simulink model "PhysicalEverSimmer"  (R2026a)
settings: Solver=VariableStepAuto  StopTime=14400
undefined symbols (not defined in the file): ES_PackRate_bph, ES_PrepRate_bph, ES_QCRate_bph, ES_Resupply_bph, Fault_T_Cell1, Fault_T_Cell2, Fault_T_Cell3, Recipe_Block_s, Recipe_Count, Resupply_Cutoff_T, Transport_Latency_s, Transport_Rate_bph
(part 1 of 2)
settings Model: DataDictionary=PhysicalEverSimmerData.sldd  Creator=sarah  LastModifiedBy=sdagen

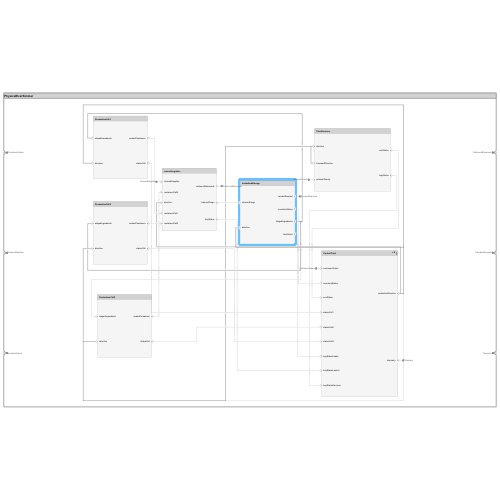
[thumbnail: Simulink's stored preview of the top-level diagram]
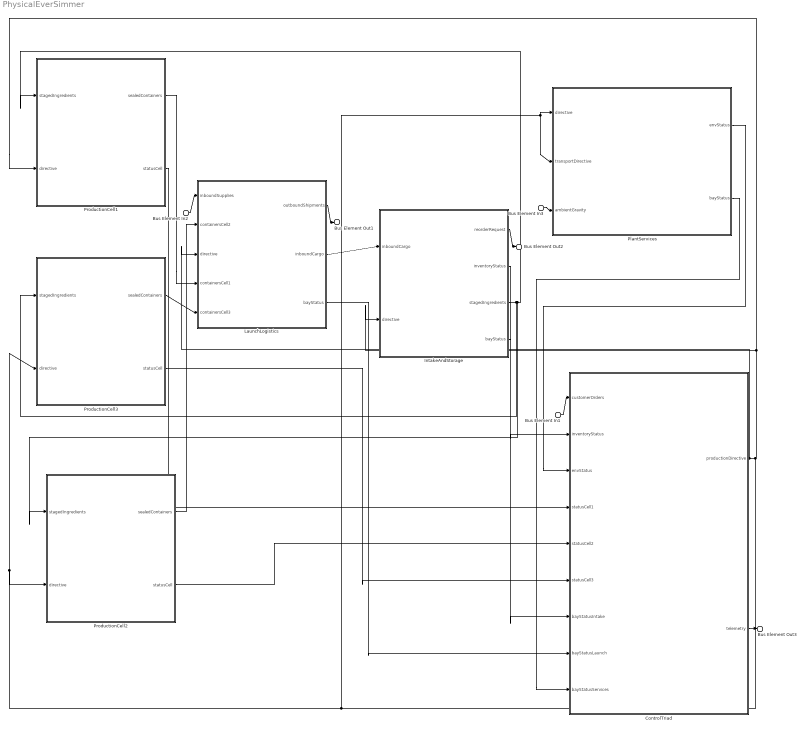
== system PhysicalEverSimmer ==
  Bus Element In1 : Inport  PortName=CustomerOrders
  Bus Element In2 : Inport  Port=2  PortName=InboundSupplies
  Bus Element In3 : Inport  Port=3  PortName=AmbientGravity
  ControlTriad : Subsystem
      settings: PortSchema="{\"entries\":[{\"content\":{\"headerSize\":26,\"margin\":15,\"minimumSpacing\":25,\"sides\":[{\"content\":{\"connectorIds\":[\"In1\",\"In2\",\"In3\",\"In4\",\"In5\",\"In6\",\"In7\",\"In8\",\"In9\"]},\"type\":\"ConnectorPlacement.EquallySpacedRectSide\",\"uuid\":\"f830f98a-8e8b-4468-adf4-d6eab644987f\"},{\"content\":{\"connectorIds\":[\"Out1\",\"Out2\"],\"side\":\"RIGHT\"},\"type\":\"ConnectorPlacement.EquallySpacedRectSide\",\"uuid\":\"7e0d0116-b3ba-4668-b638-30d0f54ba087\"},{\"content\":{\"side\":\"TOP\"},\"type\":\"ConnectorPlacement.EquallySpacedRectSide\",\"uuid\":\"7b4146d3-46d2-45ca-8c34-b106f0d8cedd\"}]},\"type\":\"ConnectorPlacement.EquallySpacedConnector\",\"uuid\":\"3d911b2d-a78f-42ea-b869-5e09982d9f54\"}],\"packageUris\":[\"http://schema.mathworks.com/mf0/Connector/R2020b\"],\"version\":\"1.0\"}"
  IntakeAndStorage : Subsystem
      settings: PortSchema="{\"entries\":[{\"content\":{\"headerSize\":26,\"margin\":15,\"minimumSpacing\":25,\"sides\":[{\"content\":{\"connectorIds\":[\"In1\",\"In2\"]},\"type\":\"ConnectorPlacement.EquallySpacedRectSide\",\"uuid\":\"3a94c7fc-0b9e-4df5-a2de-1d2483378dcb\"},{\"content\":{\"connectorIds\":[\"Out1\",\"Out2\",\"Out3\",\"Out4\"],\"side\":\"RIGHT\"},\"type\":\"ConnectorPlacement.EquallySpacedRectSide\",\"uuid\":\"607e1f04-41cc-4c9a-b401-96cdf33819d0\"},{\"content\":{\"side\":\"TOP\"},\"type\":\"ConnectorPlacement.EquallySpacedRectSide\",\"uuid\":\"2ee07fc7-54c6-4cee-9888-3f37ad01f332\"}]},\"type\":\"ConnectorPlacement.EquallySpacedConnector\",\"uuid\":\"f91f3af9-eaeb-4625-ae6e-5ceb7fb8b64c\"}],\"packageUris\":[\"http://schema.mathworks.com/mf0/Connector/R2020b\"],\"version\":\"1.0\"}"
  LaunchLogistics : Subsystem
      settings: PortSchema="{\"entries\":[{\"content\":{\"headerSize\":26,\"margin\":15,\"minimumSpacing\":25,\"sides\":[{\"content\":{\"connectorIds\":[\"In1\",\"In2\",\"In3\",\"In4\",\"In5\"]},\"type\":\"ConnectorPlacement.EquallySpacedRectSide\",\"uuid\":\"3a94c7fc-0b9e-4df5-a2de-1d2483378dcb\"},{\"content\":{\"connectorIds\":[\"Out1\",\"Out2\",\"Out3\"],\"side\":\"RIGHT\"},\"type\":\"ConnectorPlacement.EquallySpacedRectSide\",\"uuid\":\"607e1f04-41cc-4c9a-b401-96cdf33819d0\"},{\"content\":{\"side\":\"TOP\"},\"type\":\"ConnectorPlacement.EquallySpacedRectSide\",\"uuid\":\"2ee07fc7-54c6-4cee-9888-3f37ad01f332\"}]},\"type\":\"ConnectorPlacement.EquallySpacedConnector\",\"uuid\":\"f91f3af9-eaeb-4625-ae6e-5ceb7fb8b64c\"}],\"packageUris\":[\"http://schema.mathworks.com/mf0/Connector/R2020b\"],\"version\":\"1.0\"}"
  PlantServices : Subsystem
      settings: PortSchema="{\"entries\":[{\"content\":{\"headerSize\":26,\"margin\":15,\"minimumSpacing\":25,\"sides\":[{\"content\":{\"connectorIds\":[\"In1\",\"In2\",\"In3\"]},\"type\":\"ConnectorPlacement.EquallySpacedRectSide\",\"uuid\":\"3a94c7fc-0b9e-4df5-a2de-1d2483378dcb\"},{\"content\":{\"connectorIds\":[\"Out1\",\"Out2\"],\"side\":\"RIGHT\"},\"type\":\"ConnectorPlacement.EquallySpacedRectSide\",\"uuid\":\"607e1f04-41cc-4c9a-b401-96cdf33819d0\"},{\"content\":{\"side\":\"TOP\"},\"type\":\"ConnectorPlacement.EquallySpacedRectSide\",\"uuid\":\"2ee07fc7-54c6-4cee-9888-3f37ad01f332\"}]},\"type\":\"ConnectorPlacement.EquallySpacedConnector\",\"uuid\":\"f91f3af9-eaeb-4625-ae6e-5ceb7fb8b64c\"}],\"packageUris\":[\"http://schema.mathworks.com/mf0/Connector/R2020b\"],\"version\":\"1.0\"}"
  ProductionCell1 : Subsystem
      settings: PortSchema="{\"entries\":[{\"content\":{\"headerSize\":26,\"margin\":15,\"minimumSpacing\":25,\"sides\":[{\"content\":{\"connectorIds\":[\"In1\",\"In2\"]},\"type\":\"ConnectorPlacement.EquallySpacedRectSide\",\"uuid\":\"f830f98a-8e8b-4468-adf4-d6eab644987f\"},{\"content\":{\"connectorIds\":[\"Out1\",\"Out2\"],\"side\":\"RIGHT\"},\"type\":\"ConnectorPlacement.EquallySpacedRectSide\",\"uuid\":\"7e0d0116-b3ba-4668-b638-30d0f54ba087\"},{\"content\":{\"side\":\"TOP\"},\"type\":\"ConnectorPlacement.EquallySpacedRectSide\",\"uuid\":\"7b4146d3-46d2-45ca-8c34-b106f0d8cedd\"}]},\"type\":\"ConnectorPlacement.EquallySpacedConnector\",\"uuid\":\"3d911b2d-a78f-42ea-b869-5e09982d9f54\"}],\"packageUris\":[\"http://schema.mathworks.com/mf0/Connector/R2020b\"],\"version\":\"1.0\"}"
  ProductionCell2 : Subsystem
      settings: PortSchema="{\"entries\":[{\"content\":{\"headerSize\":26,\"margin\":15,\"minimumSpacing\":25,\"sides\":[{\"content\":{\"connectorIds\":[\"In1\",\"In2\"]},\"type\":\"ConnectorPlacement.EquallySpacedRectSide\",\"uuid\":\"f830f98a-8e8b-4468-adf4-d6eab644987f\"},{\"content\":{\"connectorIds\":[\"Out1\",\"Out2\"],\"side\":\"RIGHT\"},\"type\":\"ConnectorPlacement.EquallySpacedRectSide\",\"uuid\":\"7e0d0116-b3ba-4668-b638-30d0f54ba087\"},{\"content\":{\"side\":\"TOP\"},\"type\":\"ConnectorPlacement.EquallySpacedRectSide\",\"uuid\":\"7b4146d3-46d2-45ca-8c34-b106f0d8cedd\"}]},\"type\":\"ConnectorPlacement.EquallySpacedConnector\",\"uuid\":\"3d911b2d-a78f-42ea-b869-5e09982d9f54\"}],\"packageUris\":[\"http://schema.mathworks.com/mf0/Connector/R2020b\"],\"version\":\"1.0\"}"
  ProductionCell3 : Subsystem
      settings: PortSchema="{\"entries\":[{\"content\":{\"headerSize\":26,\"margin\":15,\"minimumSpacing\":25,\"sides\":[{\"content\":{\"connectorIds\":[\"In1\",\"In2\"]},\"type\":\"ConnectorPlacement.EquallySpacedRectSide\",\"uuid\":\"f830f98a-8e8b-4468-adf4-d6eab644987f\"},{\"content\":{\"connectorIds\":[\"Out1\",\"Out2\"],\"side\":\"RIGHT\"},\"type\":\"ConnectorPlacement.EquallySpacedRectSide\",\"uuid\":\"7e0d0116-b3ba-4668-b638-30d0f54ba087\"},{\"content\":{\"side\":\"TOP\"},\"type\":\"ConnectorPlacement.EquallySpacedRectSide\",\"uuid\":\"7b4146d3-46d2-45ca-8c34-b106f0d8cedd\"}]},\"type\":\"ConnectorPlacement.EquallySpacedConnector\",\"uuid\":\"3d911b2d-a78f-42ea-b869-5e09982d9f54\"}],\"packageUris\":[\"http://schema.mathworks.com/mf0/Connector/R2020b\"],\"version\":\"1.0\"}"
  Bus Element Out1 : Outport  PortName=OutboundShipments
  Bus Element Out2 : Outport  Port=2  PortName=ReorderRequests
  Bus Element Out3 : Outport  Port=3  PortName=Telemetry
  wires:
  Bus Element In2/1 -> LaunchLogistics/1(inboundSupplies)
  ProductionCell2/2(statusCell) -> ControlTriad/5(statusCell2)
  LaunchLogistics/1(outboundShipments) -> Bus Element Out1/1
  ProductionCell2/1(sealedContainers) -> LaunchLogistics/2(containersCell2)
  ProductionCell1/1(sealedContainers) -> LaunchLogistics/4(containersCell1)
  ProductionCell1/2(statusCell) -> ControlTriad/4(statusCell1)
  ProductionCell3/1(sealedContainers) -> LaunchLogistics/5(containersCell3)
  IntakeAndStorage/3(stagedIngredients) -> ProductionCell2/1(stagedIngredients), ProductionCell1/1(stagedIngredients), ProductionCell3/1(stagedIngredients)
  ProductionCell3/2(statusCell) -> ControlTriad/6(statusCell3)
  LaunchLogistics/2(inboundCargo) -> IntakeAndStorage/1(inboundCargo)
  LaunchLogistics/3(bayStatus) -> ControlTriad/8(bayStatusLaunch)
  Bus Element In3/1 -> PlantServices/3(ambientGravity)
  Bus Element In1/1 -> ControlTriad/1(customerOrders)
  IntakeAndStorage/1(reorderRequest) -> Bus Element Out2/1
  IntakeAndStorage/2(inventoryStatus) -> ControlTriad/2(inventoryStatus)
  IntakeAndStorage/4(bayStatus) -> ControlTriad/7(bayStatusIntake)
  PlantServices/1(envStatus) -> ControlTriad/3(envStatus)
  PlantServices/2(bayStatus) -> ControlTriad/9(bayStatusServices)
  ControlTriad/1(productionDirective) -> PlantServices/2(transportDirective), PlantServices/1(directive), ProductionCell3/2(directive), ProductionCell2/2(directive), IntakeAndStorage/2(directive), ProductionCell1/2(directive), LaunchLogistics/3(directive)
  ControlTriad/2(telemetry) -> Bus Element Out3/1

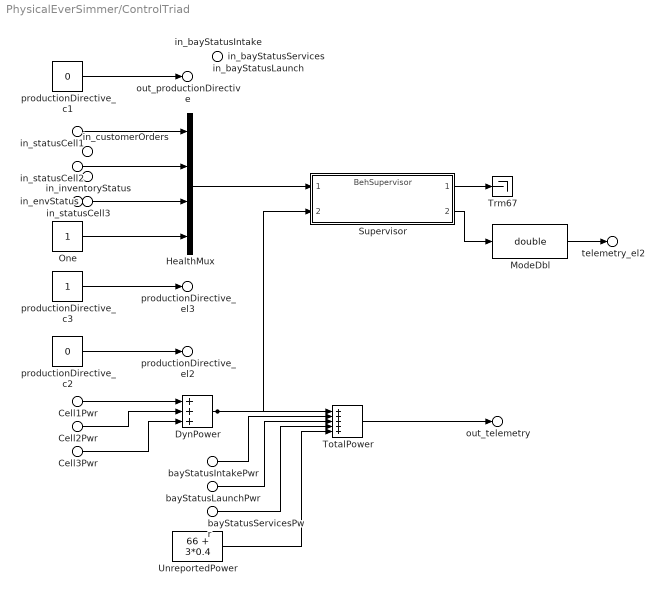
== system PhysicalEverSimmer/ControlTriad ==
  in_customerOrders : Inport  PortName=customerOrders
  in_inventoryStatus : Inport  Port=2  PortName=inventoryStatus
  in_envStatus : Inport  Port=3  PortName=envStatus
  Cell1Pwr : Inport  Port=4  PortName=statusCell1  Element=power_kW
  in_statusCell1 : Inport  Port=4  PortName=statusCell1  Element=health
  Cell2Pwr : Inport  Port=5  PortName=statusCell2  Element=power_kW
  in_statusCell2 : Inport  Port=5  PortName=statusCell2  Element=health
  Cell3Pwr : Inport  Port=6  PortName=statusCell3  Element=power_kW
  in_statusCell3 : Inport  Port=6  PortName=statusCell3  Element=health
  in_bayStatusIntake : Inport  Port=7  PortName=bayStatusIntake
  bayStatusIntakePwr : Inport  Port=7  PortName=bayStatusIntake  Element=power_kW
  in_bayStatusLaunch : Inport  Port=8  PortName=bayStatusLaunch
  bayStatusLaunchPwr : Inport  Port=8  PortName=bayStatusLaunch  Element=power_kW
  in_bayStatusServices : Inport  Port=9  PortName=bayStatusServices
  bayStatusServicesPwr : Inport  Port=9  PortName=bayStatusServices  Element=power_kW
  DynPower : Sum  Inputs=+++
  HealthMux : Mux
  ModeDbl : DataTypeConversion  OutDataTypeStr=double  SaturateOnIntegerOverflow=off  RndMeth=Floor
  One : Constant
  Supervisor : ModelReference  ModelNameDialog=BehSupervisor  ParameterArgumentNames=NumLines  ParameterArgumentValues=ES_NumLines  UsingDefaultArgumentValue=0  SimulationMode=Normal  ModelReferenceVersion=1.8
  TotalPower : Sum  Inputs=+++++
  Trm67 : Terminator
  UnreportedPower : Constant  Value=66 + 3*0.4
  productionDirective_c1 : Constant  Value=0
  productionDirective_c2 : Constant  Value=0
  productionDirective_c3 : Constant
  out_productionDirective : Outport  PortName=productionDirective  Element=cmdType
  productionDirective_el2 : Outport  PortName=productionDirective  Element=targetId
  productionDirective_el3 : Outport  PortName=productionDirective  Element=setpoint
  out_telemetry : Outport  Port=2  PortName=telemetry  Element=totalPower_kW
  telemetry_el2 : Outport  Port=2  PortName=telemetry  Element=plantMode
  wires:
  productionDirective_c1/1 -> out_productionDirective/1
  productionDirective_c2/1 -> productionDirective_el2/1
  in_statusCell3/1 -> HealthMux/3
  in_statusCell1/1 -> HealthMux/1
  in_statusCell2/1 -> HealthMux/2
  One/1 -> HealthMux/4
  productionDirective_c3/1 -> productionDirective_el3/1
  ModeDbl/1 -> telemetry_el2/1
  Cell1Pwr/1 -> DynPower/1
  bayStatusIntakePwr/1 -> TotalPower/2
  Cell2Pwr/1 -> DynPower/2
  Cell3Pwr/1 -> DynPower/3
  HealthMux/1 -> Supervisor/1
  DynPower/1 -> TotalPower/1, Supervisor/2
  bayStatusLaunchPwr/1 -> TotalPower/3
  Supervisor/1 -> Trm67/1
  bayStatusServicesPwr/1 -> TotalPower/4
  UnreportedPower/1 -> TotalPower/5
  Supervisor/2 -> ModeDbl/1
  TotalPower/1 -> out_telemetry/1

== system PhysicalEverSimmer/IntakeAndStorage ==
  Bus Element In1 : Inport  PortName=inboundCargo
  Bus Element In2 : Inport  Port=2  PortName=directive
  AutoDock : Subsystem
      settings: PortSchema="{\"entries\":[{\"content\":{\"headerSize\":26,\"margin\":15,\"minimumSpacing\":25,\"sides\":[{\"content\":{\"connectorIds\":[\"In1\",\"In2\"]},\"type\":\"ConnectorPlacement.EquallySpacedRectSide\",\"uuid\":\"f830f98a-8e8b-4468-adf4-d6eab644987f\"},{\"content\":{\"connectorIds\":[\"Out1\",\"Out2\"],\"side\":\"RIGHT\"},\"type\":\"ConnectorPlacement.EquallySpacedRectSide\",\"uuid\":\"7e0d0116-b3ba-4668-b638-30d0f54ba087\"},{\"content\":{\"side\":\"TOP\"},\"type\":\"ConnectorPlacement.EquallySpacedRectSide\",\"uuid\":\"7b4146d3-46d2-45ca-8c34-b106f0d8cedd\"}]},\"type\":\"ConnectorPlacement.EquallySpacedConnector\",\"uuid\":\"3d911b2d-a78f-42ea-b869-5e09982d9f54\"}],\"packageUris\":[\"http://schema.mathworks.com/mf0/Connector/R2020b\"],\"version\":\"1.0\"}"
  DualZoneStore : Subsystem
      settings: PortSchema="{\"entries\":[{\"content\":{\"headerSize\":26,\"margin\":15,\"minimumSpacing\":25,\"sides\":[{\"content\":{\"connectorIds\":[\"In1\",\"In2\"]},\"type\":\"ConnectorPlacement.EquallySpacedRectSide\",\"uuid\":\"f830f98a-8e8b-4468-adf4-d6eab644987f\"},{\"content\":{\"connectorIds\":[\"Out1\",\"Out2\",\"Out3\"],\"side\":\"RIGHT\"},\"type\":\"ConnectorPlacement.EquallySpacedRectSide\",\"uuid\":\"7e0d0116-b3ba-4668-b638-30d0f54ba087\"},{\"content\":{\"side\":\"TOP\"},\"type\":\"ConnectorPlacement.EquallySpacedRectSide\",\"uuid\":\"7b4146d3-46d2-45ca-8c34-b106f0d8cedd\"}]},\"type\":\"ConnectorPlacement.EquallySpacedConnector\",\"uuid\":\"3d911b2d-a78f-42ea-b869-5e09982d9f54\"}],\"packageUris\":[\"http://schema.mathworks.com/mf0/Connector/R2020b\"],\"version\":\"1.0\"}"
  IntakeController : Subsystem
      settings: PortSchema="{\"entries\":[{\"content\":{\"headerSize\":26,\"margin\":15,\"minimumSpacing\":25,\"sides\":[{\"content\":{\"connectorIds\":[\"In1\",\"In2\",\"In3\"]},\"type\":\"ConnectorPlacement.EquallySpacedRectSide\",\"uuid\":\"0731d988-4a26-4db6-8347-b78d2aa6954f\"},{\"content\":{\"connectorIds\":[\"Out1\",\"Out2\"],\"side\":\"RIGHT\"},\"type\":\"ConnectorPlacement.EquallySpacedRectSide\",\"uuid\":\"6e8ac7ed-a816-4c7e-8f31-c61224c9ac03\"},{\"content\":{\"side\":\"TOP\"},\"type\":\"ConnectorPlacement.EquallySpacedRectSide\",\"uuid\":\"7c48a918-2743-4697-bc21-ce4fb8bbcea2\"}]},\"type\":\"ConnectorPlacement.EquallySpacedConnector\",\"uuid\":\"5e30be34-c1af-4919-9af8-d4df8145ecd1\"}],\"packageUris\":[\"http://schema.mathworks.com/mf0/Connector/R2020b\"],\"version\":\"1.0\"}"
  SmartInventoryNet : Subsystem
      settings: PortSchema="{\"entries\":[{\"content\":{\"headerSize\":26,\"margin\":15,\"minimumSpacing\":25,\"sides\":[{\"content\":{\"connectorIds\":[\"In1\"]},\"type\":\"ConnectorPlacement.EquallySpacedRectSide\",\"uuid\":\"f830f98a-8e8b-4468-adf4-d6eab644987f\"},{\"content\":{\"connectorIds\":[\"Out1\",\"Out2\"],\"side\":\"RIGHT\"},\"type\":\"ConnectorPlacement.EquallySpacedRectSide\",\"uuid\":\"7e0d0116-b3ba-4668-b638-30d0f54ba087\"},{\"content\":{\"side\":\"TOP\"},\"type\":\"ConnectorPlacement.EquallySpacedRectSide\",\"uuid\":\"7b4146d3-46d2-45ca-8c34-b106f0d8cedd\"}]},\"type\":\"ConnectorPlacement.EquallySpacedConnector\",\"uuid\":\"3d911b2d-a78f-42ea-b869-5e09982d9f54\"}],\"packageUris\":[\"http://schema.mathworks.com/mf0/Connector/R2020b\"],\"version\":\"1.0\"}"
  Bus Element Out1 : Outport  PortName=reorderRequest
  Bus Element Out2 : Outport  Port=2  PortName=inventoryStatus
  Bus Element Out3 : Outport  Port=3  PortName=stagedIngredients
  Bus Element Out6 : Outport  Port=4  PortName=bayStatus
  wires:
  DualZoneStore/1(stagedIngredients) -> Bus Element Out3/1
  AutoDock/1(receivedIngredients) -> DualZoneStore/1(receivedIngredients)
  Bus Element In2/1 -> IntakeController/1(directive)
  DualZoneStore/3(statusStore) -> IntakeController/3(statusStore)
  Bus Element In1/1 -> AutoDock/1(inboundCargo)
  IntakeController/1(bayDirective) -> DualZoneStore/2(directive), AutoDock/2(directive)
  IntakeController/2(bayStatus) -> Bus Element Out6/1
  DualZoneStore/2(stockLevel) -> SmartInventoryNet/1(stockLevel)
  AutoDock/2(statusReceive) -> IntakeController/2(statusReceive)
  SmartInventoryNet/1(inventoryStatus) -> Bus Element Out2/1
  SmartInventoryNet/2(reorderRequest) -> Bus Element Out1/1

== system PhysicalEverSimmer/LaunchLogistics ==
  Bus Element In1 : Inport  PortName=inboundSupplies
  Bus Element In2 : Inport  Port=2  PortName=containersCell2
  Bus Element In3 : Inport  Port=3  PortName=directive
  Bus Element In4 : Inport  Port=4  PortName=containersCell1
  Bus Element In7 : Inport  Port=5  PortName=containersCell3
  AutoCargoLoader : Subsystem
      settings: PortSchema="{\"entries\":[{\"content\":{\"headerSize\":26,\"margin\":15,\"minimumSpacing\":25,\"sides\":[{\"content\":{\"connectorIds\":[\"In1\",\"In2\",\"In3\",\"In4\"]},\"type\":\"ConnectorPlacement.EquallySpacedRectSide\",\"uuid\":\"f830f98a-8e8b-4468-adf4-d6eab644987f\"},{\"content\":{\"connectorIds\":[\"Out1\",\"Out2\",\"Out3\"],\"side\":\"RIGHT\"},\"type\":\"ConnectorPlacement.EquallySpacedRectSide\",\"uuid\":\"7e0d0116-b3ba-4668-b638-30d0f54ba087\"},{\"content\":{\"side\":\"TOP\"},\"type\":\"ConnectorPlacement.EquallySpacedRectSide\",\"uuid\":\"7b4146d3-46d2-45ca-8c34-b106f0d8cedd\"}]},\"type\":\"ConnectorPlacement.EquallySpacedConnector\",\"uuid\":\"3d911b2d-a78f-42ea-b869-5e09982d9f54\"}],\"packageUris\":[\"http://schema.mathworks.com/mf0/Connector/R2020b\"],\"version\":\"1.0\"}"
  AutoRefuelCell : Subsystem
      settings: PortSchema="{\"entries\":[{\"content\":{\"headerSize\":26,\"margin\":15,\"minimumSpacing\":25,\"sides\":[{\"content\":{\"connectorIds\":[\"In1\"]},\"type\":\"ConnectorPlacement.EquallySpacedRectSide\",\"uuid\":\"f830f98a-8e8b-4468-adf4-d6eab644987f\"},{\"content\":{\"connectorIds\":[\"Out1\"],\"side\":\"RIGHT\"},\"type\":\"ConnectorPlacement.EquallySpacedRectSide\",\"uuid\":\"7e0d0116-b3ba-4668-b638-30d0f54ba087\"},{\"content\":{\"side\":\"TOP\"},\"type\":\"ConnectorPlacement.EquallySpacedRectSide\",\"uuid\":\"7b4146d3-46d2-45ca-8c34-b106f0d8cedd\"}]},\"type\":\"ConnectorPlacement.EquallySpacedConnector\",\"uuid\":\"3d911b2d-a78f-42ea-b869-5e09982d9f54\"}],\"packageUris\":[\"http://schema.mathworks.com/mf0/Connector/R2020b\"],\"version\":\"1.0\"}"
  LaunchController : Subsystem
      settings: PortSchema="{\"entries\":[{\"content\":{\"headerSize\":26,\"margin\":15,\"minimumSpacing\":25,\"sides\":[{\"content\":{\"connectorIds\":[\"In1\",\"In2\",\"In3\",\"In4\"]},\"type\":\"ConnectorPlacement.EquallySpacedRectSide\",\"uuid\":\"0731d988-4a26-4db6-8347-b78d2aa6954f\"},{\"content\":{\"connectorIds\":[\"Out1\",\"Out2\"],\"side\":\"RIGHT\"},\"type\":\"ConnectorPlacement.EquallySpacedRectSide\",\"uuid\":\"6e8ac7ed-a816-4c7e-8f31-c61224c9ac03\"},{\"content\":{\"side\":\"TOP\"},\"type\":\"ConnectorPlacement.EquallySpacedRectSide\",\"uuid\":\"7c48a918-2743-4697-bc21-ce4fb8bbcea2\"}]},\"type\":\"ConnectorPlacement.EquallySpacedConnector\",\"uuid\":\"5e30be34-c1af-4919-9af8-d4df8145ecd1\"}],\"packageUris\":[\"http://schema.mathworks.com/mf0/Connector/R2020b\"],\"version\":\"1.0\"}"
  TriplePadPort : Subsystem
      settings: PortSchema="{\"entries\":[{\"content\":{\"headerSize\":26,\"margin\":15,\"minimumSpacing\":25,\"sides\":[{\"content\":{\"connectorIds\":[\"In1\",\"In2\",\"In3\",\"In4\"]},\"type\":\"ConnectorPlacement.EquallySpacedRectSide\",\"uuid\":\"f830f98a-8e8b-4468-adf4-d6eab644987f\"},{\"content\":{\"connectorIds\":[\"Out1\",\"Out2\",\"Out3\"],\"side\":\"RIGHT\"},\"type\":\"ConnectorPlacement.EquallySpacedRectSide\",\"uuid\":\"7e0d0116-b3ba-4668-b638-30d0f54ba087\"},{\"content\":{\"side\":\"TOP\"},\"type\":\"ConnectorPlacement.EquallySpacedRectSide\",\"uuid\":\"7b4146d3-46d2-45ca-8c34-b106f0d8cedd\"}]},\"type\":\"ConnectorPlacement.EquallySpacedConnector\",\"uuid\":\"3d911b2d-a78f-42ea-b869-5e09982d9f54\"}],\"packageUris\":[\"http://schema.mathworks.com/mf0/Connector/R2020b\"],\"version\":\"1.0\"}"
  Bus Element Out1 : Outport  PortName=outboundShipments
  Bus Element Out2 : Outport  Port=2  PortName=inboundCargo
  Bus Element Out6 : Outport  Port=3  PortName=bayStatus
  wires:
  Bus Element In7/1 -> AutoCargoLoader/3(containersCell3)
  Bus Element In3/1 -> LaunchController/1(directive)
  Bus Element In1/1 -> TriplePadPort/4(inboundSupplies)
  TriplePadPort/1(inboundCargo) -> Bus Element Out2/1
  TriplePadPort/2(outboundShipments) -> Bus Element Out1/1
  AutoRefuelCell/1(statusRefuel) -> LaunchController/3(statusRefuel)
  TriplePadPort/3(statusFleet) -> LaunchController/4(statusFleet)
  Bus Element In2/1 -> AutoCargoLoader/2(containersCell2)
  Bus Element In4/1 -> AutoCargoLoader/1(containersCell1)
  LaunchController/1(bayDirective) -> TriplePadPort/3(directive), AutoRefuelCell/1(directive), AutoCargoLoader/4(directive)
  LaunchController/2(bayStatus) -> Bus Element Out6/1
  AutoCargoLoader/1(loadedShipment) -> TriplePadPort/1(loadedShipment)
  AutoCargoLoader/2(manifest) -> TriplePadPort/2(manifest)
  AutoCargoLoader/3(statusDispatch) -> LaunchController/2(statusDispatch)

== system PhysicalEverSimmer/PlantServices ==
  Bus Element In1 : Inport  PortName=directive
  Bus Element In2 : Inport  Port=2  PortName=transportDirective
  Bus Element In3 : Inport  Port=3  PortName=ambientGravity
  GravityCompMesh : Subsystem
      settings: PortSchema="{\"entries\":[{\"content\":{\"headerSize\":26,\"margin\":15,\"minimumSpacing\":25,\"sides\":[{\"content\":{\"connectorIds\":[\"In1\"]},\"type\":\"ConnectorPlacement.EquallySpacedRectSide\",\"uuid\":\"f830f98a-8e8b-4468-adf4-d6eab644987f\"},{\"content\":{\"connectorIds\":[\"Out1\"],\"side\":\"RIGHT\"},\"type\":\"ConnectorPlacement.EquallySpacedRectSide\",\"uuid\":\"7e0d0116-b3ba-4668-b638-30d0f54ba087\"},{\"content\":{\"side\":\"TOP\"},\"type\":\"ConnectorPlacement.EquallySpacedRectSide\",\"uuid\":\"7b4146d3-46d2-45ca-8c34-b106f0d8cedd\"}]},\"type\":\"ConnectorPlacement.EquallySpacedConnector\",\"uuid\":\"3d911b2d-a78f-42ea-b869-5e09982d9f54\"}],\"packageUris\":[\"http://schema.mathworks.com/mf0/Connector/R2020b\"],\"version\":\"1.0\"}"
  RedundantReactorPair : Subsystem
      settings: PortSchema="{\"entries\":[{\"content\":{\"headerSize\":26,\"margin\":15,\"minimumSpacing\":25,\"sides\":[{\"content\":{\"connectorIds\":[\"In1\"]},\"type\":\"ConnectorPlacement.EquallySpacedRectSide\",\"uuid\":\"f830f98a-8e8b-4468-adf4-d6eab644987f\"},{\"content\":{\"connectorIds\":[\"Out1\"],\"side\":\"RIGHT\"},\"type\":\"ConnectorPlacement.EquallySpacedRectSide\",\"uuid\":\"7e0d0116-b3ba-4668-b638-30d0f54ba087\"},{\"content\":{\"side\":\"TOP\"},\"type\":\"ConnectorPlacement.EquallySpacedRectSide\",\"uuid\":\"7b4146d3-46d2-45ca-8c34-b106f0d8cedd\"}]},\"type\":\"ConnectorPlacement.EquallySpacedConnector\",\"uuid\":\"3d911b2d-a78f-42ea-b869-5e09982d9f54\"}],\"packageUris\":[\"http://schema.mathworks.com/mf0/Connector/R2020b\"],\"version\":\"1.0\"}"
  RoboTransportSwarm : Subsystem
      settings: PortSchema="{\"entries\":[{\"content\":{\"headerSize\":26,\"margin\":15,\"minimumSpacing\":25,\"sides\":[{\"content\":{\"connectorIds\":[\"In1\"]},\"type\":\"ConnectorPlacement.EquallySpacedRectSide\",\"uuid\":\"f830f98a-8e8b-4468-adf4-d6eab644987f\"},{\"content\":{\"connectorIds\":[\"Out1\"],\"side\":\"RIGHT\"},\"type\":\"ConnectorPlacement.EquallySpacedRectSide\",\"uuid\":\"7e0d0116-b3ba-4668-b638-30d0f54ba087\"},{\"content\":{\"side\":\"TOP\"},\"type\":\"ConnectorPlacement.EquallySpacedRectSide\",\"uuid\":\"7b4146d3-46d2-45ca-8c34-b106f0d8cedd\"}]},\"type\":\"ConnectorPlacement.EquallySpacedConnector\",\"uuid\":\"3d911b2d-a78f-42ea-b869-5e09982d9f54\"}],\"packageUris\":[\"http://schema.mathworks.com/mf0/Connector/R2020b\"],\"version\":\"1.0\"}"
  ServicesController : Subsystem
      settings: PortSchema="{\"entries\":[{\"content\":{\"headerSize\":26,\"margin\":15,\"minimumSpacing\":25,\"sides\":[{\"content\":{\"connectorIds\":[\"In1\",\"In2\",\"In3\"]},\"type\":\"ConnectorPlacement.EquallySpacedRectSide\",\"uuid\":\"0731d988-4a26-4db6-8347-b78d2aa6954f\"},{\"content\":{\"connectorIds\":[\"Out1\",\"Out2\"],\"side\":\"RIGHT\"},\"type\":\"ConnectorPlacement.EquallySpacedRectSide\",\"uuid\":\"6e8ac7ed-a816-4c7e-8f31-c61224c9ac03\"},{\"content\":{\"side\":\"TOP\"},\"type\":\"ConnectorPlacement.EquallySpacedRectSide\",\"uuid\":\"7c48a918-2743-4697-bc21-ce4fb8bbcea2\"}]},\"type\":\"ConnectorPlacement.EquallySpacedConnector\",\"uuid\":\"5e30be34-c1af-4919-9af8-d4df8145ecd1\"}],\"packageUris\":[\"http://schema.mathworks.com/mf0/Connector/R2020b\"],\"version\":\"1.0\"}"
  Bus Element Out1 : Outport  PortName=envStatus
  Bus Element Out4 : Outport  Port=2  PortName=bayStatus
  wires:
  RedundantReactorPair/1(statusPower) -> ServicesController/2(statusPower)
  Bus Element In1/1 -> ServicesController/1(directive)
  Bus Element In3/1 -> GravityCompMesh/1(ambientGravity)
  ServicesController/1(bayDirective) -> RedundantReactorPair/1(directive)
  RoboTransportSwarm/1(statusTransport) -> ServicesController/3(statusTransport)
  Bus Element In2/1 -> RoboTransportSwarm/1(transportDirective)
  ServicesController/2(bayStatus) -> Bus Element Out4/1
  GravityCompMesh/1(envStatus) -> Bus Element Out1/1

== system PhysicalEverSimmer/ProductionCell1 ==
  Bus Element In1 : Inport  PortName=stagedIngredients
  Bus Element In2 : Inport  Port=2  PortName=directive
  CellController : Subsystem
      settings: PortSchema="{\"entries\":[{\"content\":{\"headerSize\":26,\"margin\":15,\"minimumSpacing\":25,\"sides\":[{\"content\":{\"connectorIds\":[\"In1\",\"In2\",\"In3\",\"In4\",\"In5\"]},\"type\":\"ConnectorPlacement.EquallySpacedRectSide\",\"uuid\":\"f830f98a-8e8b-4468-adf4-d6eab644987f\"},{\"content\":{\"connectorIds\":[\"Out1\",\"Out2\"],\"side\":\"RIGHT\"},\"type\":\"ConnectorPlacement.EquallySpacedRectSide\",\"uuid\":\"7e0d0116-b3ba-4668-b638-30d0f54ba087\"},{\"content\":{\"side\":\"TOP\"},\"type\":\"ConnectorPlacement.EquallySpacedRectSide\",\"uuid\":\"7b4146d3-46d2-45ca-8c34-b106f0d8cedd\"}]},\"type\":\"ConnectorPlacement.EquallySpacedConnector\",\"uuid\":\"3d911b2d-a78f-42ea-b869-5e09982d9f54\"}],\"packageUris\":[\"http://schema.mathworks.com/mf0/Connector/R2020b\"],\"version\":\"1.0\"}"
  CellCookVat : Subsystem
      settings: PortSchema="{\"entries\":[{\"content\":{\"headerSize\":26,\"margin\":15,\"minimumSpacing\":25,\"sides\":[{\"content\":{\"connectorIds\":[\"In1\",\"In2\"]},\"type\":\"ConnectorPlacement.EquallySpacedRectSide\",\"uuid\":\"f830f98a-8e8b-4468-adf4-d6eab644987f\"},{\"content\":{\"connectorIds\":[\"Out1\",\"Out2\"],\"side\":\"RIGHT\"},\"type\":\"ConnectorPlacement.EquallySpacedRectSide\",\"uuid\":\"7e0d0116-b3ba-4668-b638-30d0f54ba087\"},{\"content\":{\"side\":\"TOP\"},\"type\":\"ConnectorPlacement.EquallySpacedRectSide\",\"uuid\":\"7b4146d3-46d2-45ca-8c34-b106f0d8cedd\"}]},\"type\":\"ConnectorPlacement.EquallySpacedConnector\",\"uuid\":\"3d911b2d-a78f-42ea-b869-5e09982d9f54\"}],\"packageUris\":[\"http://schema.mathworks.com/mf0/Connector/R2020b\"],\"version\":\"1.0\"}"
  CellPackager : Subsystem
      settings: PortSchema="{\"entries\":[{\"content\":{\"headerSize\":26,\"margin\":15,\"minimumSpacing\":25,\"sides\":[{\"content\":{\"connectorIds\":[\"In1\",\"In2\"]},\"type\":\"ConnectorPlacement.EquallySpacedRectSide\",\"uuid\":\"f830f98a-8e8b-4468-adf4-d6eab644987f\"},{\"content\":{\"connectorIds\":[\"Out1\",\"Out2\"],\"side\":\"RIGHT\"},\"type\":\"ConnectorPlacement.EquallySpacedRectSide\",\"uuid\":\"7e0d0116-b3ba-4668-b638-30d0f54ba087\"},{\"content\":{\"side\":\"TOP\"},\"type\":\"ConnectorPlacement.EquallySpacedRectSide\",\"uuid\":\"7b4146d3-46d2-45ca-8c34-b106f0d8cedd\"}]},\"type\":\"ConnectorPlacement.EquallySpacedConnector\",\"uuid\":\"3d911b2d-a78f-42ea-b869-5e09982d9f54\"}],\"packageUris\":[\"http://schema.mathworks.com/mf0/Connector/R2020b\"],\"version\":\"1.0\"}"
  CellPrepUnit : Subsystem
      settings: PortSchema="{\"entries\":[{\"content\":{\"headerSize\":26,\"margin\":15,\"minimumSpacing\":25,\"sides\":[{\"content\":{\"connectorIds\":[\"In1\",\"In2\"]},\"type\":\"ConnectorPlacement.EquallySpacedRectSide\",\"uuid\":\"f830f98a-8e8b-4468-adf4-d6eab644987f\"},{\"content\":{\"connectorIds\":[\"Out1\",\"Out2\"],\"side\":\"RIGHT\"},\"type\":\"ConnectorPlacement.EquallySpacedRectSide\",\"uuid\":\"7e0d0116-b3ba-4668-b638-30d0f54ba087\"},{\"content\":{\"side\":\"TOP\"},\"type\":\"ConnectorPlacement.EquallySpacedRectSide\",\"uuid\":\"7b4146d3-46d2-45ca-8c34-b106f0d8cedd\"}]},\"type\":\"ConnectorPlacement.EquallySpacedConnector\",\"uuid\":\"3d911b2d-a78f-42ea-b869-5e09982d9f54\"}],\"packageUris\":[\"http://schema.mathworks.com/mf0/Connector/R2020b\"],\"version\":\"1.0\"}"
  CellQCSensor : Subsystem
      settings: PortSchema="{\"entries\":[{\"content\":{\"headerSize\":26,\"margin\":15,\"minimumSpacing\":25,\"sides\":[{\"content\":{\"connectorIds\":[\"In1\",\"In2\"]},\"type\":\"ConnectorPlacement.EquallySpacedRectSide\",\"uuid\":\"f830f98a-8e8b-4468-adf4-d6eab644987f\"},{\"content\":{\"connectorIds\":[\"Out1\",\"Out2\"],\"side\":\"RIGHT\"},\"type\":\"ConnectorPlacement.EquallySpacedRectSide\",\"uuid\":\"7e0d0116-b3ba-4668-b638-30d0f54ba087\"},{\"content\":{\"side\":\"TOP\"},\"type\":\"ConnectorPlacement.EquallySpacedRectSide\",\"uuid\":\"7b4146d3-46d2-45ca-8c34-b106f0d8cedd\"}]},\"type\":\"ConnectorPlacement.EquallySpacedConnector\",\"uuid\":\"3d911b2d-a78f-42ea-b869-5e09982d9f54\"}],\"packageUris\":[\"http://schema.mathworks.com/mf0/Connector/R2020b\"],\"version\":\"1.0\"}"
  Bus Element Out1 : Outport  PortName=sealedContainers
  Bus Element Out2 : Outport  Port=2  PortName=statusCell
  wires:
  CellPackager/1(sealedContainers) -> Bus Element Out1/1
  Bus Element In1/1 -> CellPrepUnit/1(stagedIngredients)
  CellQCSensor/1(approvedSoup) -> CellPackager/1(approvedSoup)
  CellQCSensor/2(statusQA) -> CellController/4(statusQA)
  CellPackager/2(statusPack) -> CellController/5(statusPack)
  CellPrepUnit/1(preppedBatch) -> CellCookVat/1(preppedBatch)
  CellPrepUnit/2(statusPrep) -> CellController/2(statusPrep)
  CellCookVat/1(cookedSoup) -> CellQCSensor/1(cookedSoup)
  CellCookVat/2(statusCook) -> CellController/3(statusCook)
  Bus Element In2/1 -> CellController/1(directive)
  CellController/1(cellDirective) -> CellQCSensor/2(directive), CellPackager/2(directive), CellCookVat/2(directive), CellPrepUnit/2(directive)
  CellController/2(statusCell) -> Bus Element Out2/1

== system PhysicalEverSimmer/ProductionCell2 ==
  Bus Element In1 : Inport  PortName=stagedIngredients
  Bus Element In2 : Inport  Port=2  PortName=directive
  CellController : Subsystem
      settings: PortSchema="{\"entries\":[{\"content\":{\"headerSize\":26,\"margin\":15,\"minimumSpacing\":25,\"sides\":[{\"content\":{\"connectorIds\":[\"In1\",\"In2\",\"In3\",\"In4\",\"In5\"]},\"type\":\"ConnectorPlacement.EquallySpacedRectSide\",\"uuid\":\"f830f98a-8e8b-4468-adf4-d6eab644987f\"},{\"content\":{\"connectorIds\":[\"Out1\",\"Out2\"],\"side\":\"RIGHT\"},\"type\":\"ConnectorPlacement.EquallySpacedRectSide\",\"uuid\":\"7e0d0116-b3ba-4668-b638-30d0f54ba087\"},{\"content\":{\"side\":\"TOP\"},\"type\":\"ConnectorPlacement.EquallySpacedRectSide\",\"uuid\":\"7b4146d3-46d2-45ca-8c34-b106f0d8cedd\"}]},\"type\":\"ConnectorPlacement.EquallySpacedConnector\",\"uuid\":\"3d911b2d-a78f-42ea-b869-5e09982d9f54\"}],\"packageUris\":[\"http://schema.mathworks.com/mf0/Connector/R2020b\"],\"version\":\"1.0\"}"
  CellCookVat : Subsystem
      settings: PortSchema="{\"entries\":[{\"content\":{\"headerSize\":26,\"margin\":15,\"minimumSpacing\":25,\"sides\":[{\"content\":{\"connectorIds\":[\"In1\",\"In2\"]},\"type\":\"ConnectorPlacement.EquallySpacedRectSide\",\"uuid\":\"f830f98a-8e8b-4468-adf4-d6eab644987f\"},{\"content\":{\"connectorIds\":[\"Out1\",\"Out2\"],\"side\":\"RIGHT\"},\"type\":\"ConnectorPlacement.EquallySpacedRectSide\",\"uuid\":\"7e0d0116-b3ba-4668-b638-30d0f54ba087\"},{\"content\":{\"side\":\"TOP\"},\"type\":\"ConnectorPlacement.EquallySpacedRectSide\",\"uuid\":\"7b4146d3-46d2-45ca-8c34-b106f0d8cedd\"}]},\"type\":\"ConnectorPlacement.EquallySpacedConnector\",\"uuid\":\"3d911b2d-a78f-42ea-b869-5e09982d9f54\"}],\"packageUris\":[\"http://schema.mathworks.com/mf0/Connector/R2020b\"],\"version\":\"1.0\"}"
  CellPackager : Subsystem
      settings: PortSchema="{\"entries\":[{\"content\":{\"headerSize\":26,\"margin\":15,\"minimumSpacing\":25,\"sides\":[{\"content\":{\"connectorIds\":[\"In1\",\"In2\"]},\"type\":\"ConnectorPlacement.EquallySpacedRectSide\",\"uuid\":\"f830f98a-8e8b-4468-adf4-d6eab644987f\"},{\"content\":{\"connectorIds\":[\"Out1\",\"Out2\"],\"side\":\"RIGHT\"},\"type\":\"ConnectorPlacement.EquallySpacedRectSide\",\"uuid\":\"7e0d0116-b3ba-4668-b638-30d0f54ba087\"},{\"content\":{\"side\":\"TOP\"},\"type\":\"ConnectorPlacement.EquallySpacedRectSide\",\"uuid\":\"7b4146d3-46d2-45ca-8c34-b106f0d8cedd\"}]},\"type\":\"ConnectorPlacement.EquallySpacedConnector\",\"uuid\":\"3d911b2d-a78f-42ea-b869-5e09982d9f54\"}],\"packageUris\":[\"http://schema.mathworks.com/mf0/Connector/R2020b\"],\"version\":\"1.0\"}"
  CellPrepUnit : Subsystem
      settings: PortSchema="{\"entries\":[{\"content\":{\"headerSize\":26,\"margin\":15,\"minimumSpacing\":25,\"sides\":[{\"content\":{\"connectorIds\":[\"In1\",\"In2\"]},\"type\":\"ConnectorPlacement.EquallySpacedRectSide\",\"uuid\":\"f830f98a-8e8b-4468-adf4-d6eab644987f\"},{\"content\":{\"connectorIds\":[\"Out1\",\"Out2\"],\"side\":\"RIGHT\"},\"type\":\"ConnectorPlacement.EquallySpacedRectSide\",\"uuid\":\"7e0d0116-b3ba-4668-b638-30d0f54ba087\"},{\"content\":{\"side\":\"TOP\"},\"type\":\"ConnectorPlacement.EquallySpacedRectSide\",\"uuid\":\"7b4146d3-46d2-45ca-8c34-b106f0d8cedd\"}]},\"type\":\"ConnectorPlacement.EquallySpacedConnector\",\"uuid\":\"3d911b2d-a78f-42ea-b869-5e09982d9f54\"}],\"packageUris\":[\"http://schema.mathworks.com/mf0/Connector/R2020b\"],\"version\":\"1.0\"}"
  CellQCSensor : Subsystem
      settings: PortSchema="{\"entries\":[{\"content\":{\"headerSize\":26,\"margin\":15,\"minimumSpacing\":25,\"sides\":[{\"content\":{\"connectorIds\":[\"In1\",\"In2\"]},\"type\":\"ConnectorPlacement.EquallySpacedRectSide\",\"uuid\":\"f830f98a-8e8b-4468-adf4-d6eab644987f\"},{\"content\":{\"connectorIds\":[\"Out1\",\"Out2\"],\"side\":\"RIGHT\"},\"type\":\"ConnectorPlacement.EquallySpacedRectSide\",\"uuid\":\"7e0d0116-b3ba-4668-b638-30d0f54ba087\"},{\"content\":{\"side\":\"TOP\"},\"type\":\"ConnectorPlacement.EquallySpacedRectSide\",\"uuid\":\"7b4146d3-46d2-45ca-8c34-b106f0d8cedd\"}]},\"type\":\"ConnectorPlacement.EquallySpacedConnector\",\"uuid\":\"3d911b2d-a78f-42ea-b869-5e09982d9f54\"}],\"packageUris\":[\"http://schema.mathworks.com/mf0/Connector/R2020b\"],\"version\":\"1.0\"}"
  Bus Element Out1 : Outport  PortName=sealedContainers
  Bus Element Out2 : Outport  Port=2  PortName=statusCell
  wires:
  Bus Element In1/1 -> CellPrepUnit/1(stagedIngredients)
  CellQCSensor/1(approvedSoup) -> CellPackager/1(approvedSoup)
  CellPrepUnit/1(preppedBatch) -> CellCookVat/1(preppedBatch)
  CellCookVat/1(cookedSoup) -> CellQCSensor/1(cookedSoup)
  CellQCSensor/2(statusQA) -> CellController/4(statusQA)
  CellPrepUnit/2(statusPrep) -> CellController/2(statusPrep)
  CellCookVat/2(statusCook) -> CellController/3(statusCook)
  Bus Element In2/1 -> CellController/1(directive)
  CellPackager/1(sealedContainers) -> Bus Element Out1/1
  CellPackager/2(statusPack) -> CellController/5(statusPack)
  CellController/1(cellDirective) -> CellQCSensor/2(directive), CellPackager/2(directive), CellCookVat/2(directive), CellPrepUnit/2(directive)
  CellController/2(statusCell) -> Bus Element Out2/1

== system PhysicalEverSimmer/ProductionCell3 ==
  Bus Element In1 : Inport  PortName=stagedIngredients
  Bus Element In2 : Inport  Port=2  PortName=directive
  CellController : Subsystem
      settings: PortSchema="{\"entries\":[{\"content\":{\"headerSize\":26,\"margin\":15,\"minimumSpacing\":25,\"sides\":[{\"content\":{\"connectorIds\":[\"In1\",\"In2\",\"In3\",\"In4\",\"In5\"]},\"type\":\"ConnectorPlacement.EquallySpacedRectSide\",\"uuid\":\"f830f98a-8e8b-4468-adf4-d6eab644987f\"},{\"content\":{\"connectorIds\":[\"Out1\",\"Out2\"],\"side\":\"RIGHT\"},\"type\":\"ConnectorPlacement.EquallySpacedRectSide\",\"uuid\":\"7e0d0116-b3ba-4668-b638-30d0f54ba087\"},{\"content\":{\"side\":\"TOP\"},\"type\":\"ConnectorPlacement.EquallySpacedRectSide\",\"uuid\":\"7b4146d3-46d2-45ca-8c34-b106f0d8cedd\"}]},\"type\":\"ConnectorPlacement.EquallySpacedConnector\",\"uuid\":\"3d911b2d-a78f-42ea-b869-5e09982d9f54\"}],\"packageUris\":[\"http://schema.mathworks.com/mf0/Connector/R2020b\"],\"version\":\"1.0\"}"
  CellCookVat : Subsystem
      settings: PortSchema="{\"entries\":[{\"content\":{\"headerSize\":26,\"margin\":15,\"minimumSpacing\":25,\"sides\":[{\"content\":{\"connectorIds\":[\"In1\",\"In2\"]},\"type\":\"ConnectorPlacement.EquallySpacedRectSide\",\"uuid\":\"f830f98a-8e8b-4468-adf4-d6eab644987f\"},{\"content\":{\"connectorIds\":[\"Out1\",\"Out2\"],\"side\":\"RIGHT\"},\"type\":\"ConnectorPlacement.EquallySpacedRectSide\",\"uuid\":\"7e0d0116-b3ba-4668-b638-30d0f54ba087\"},{\"content\":{\"side\":\"TOP\"},\"type\":\"ConnectorPlacement.EquallySpacedRectSide\",\"uuid\":\"7b4146d3-46d2-45ca-8c34-b106f0d8cedd\"}]},\"type\":\"ConnectorPlacement.EquallySpacedConnector\",\"uuid\":\"3d911b2d-a78f-42ea-b869-5e09982d9f54\"}],\"packageUris\":[\"http://schema.mathworks.com/mf0/Connector/R2020b\"],\"version\":\"1.0\"}"
  CellPackager : Subsystem
      settings: PortSchema="{\"entries\":[{\"content\":{\"headerSize\":26,\"margin\":15,\"minimumSpacing\":25,\"sides\":[{\"content\":{\"connectorIds\":[\"In1\",\"In2\"]},\"type\":\"ConnectorPlacement.EquallySpacedRectSide\",\"uuid\":\"f830f98a-8e8b-4468-adf4-d6eab644987f\"},{\"content\":{\"connectorIds\":[\"Out1\",\"Out2\"],\"side\":\"RIGHT\"},\"type\":\"ConnectorPlacement.EquallySpacedRectSide\",\"uuid\":\"7e0d0116-b3ba-4668-b638-30d0f54ba087\"},{\"content\":{\"side\":\"TOP\"},\"type\":\"ConnectorPlacement.EquallySpacedRectSide\",\"uuid\":\"7b4146d3-46d2-45ca-8c34-b106f0d8cedd\"}]},\"type\":\"ConnectorPlacement.EquallySpacedConnector\",\"uuid\":\"3d911b2d-a78f-42ea-b869-5e09982d9f54\"}],\"packageUris\":[\"http://schema.mathworks.com/mf0/Connector/R2020b\"],\"version\":\"1.0\"}"
  CellPrepUnit : Subsystem
      settings: PortSchema="{\"entries\":[{\"content\":{\"headerSize\":26,\"margin\":15,\"minimumSpacing\":25,\"sides\":[{\"content\":{\"connectorIds\":[\"In1\",\"In2\"]},\"type\":\"ConnectorPlacement.EquallySpacedRectSide\",\"uuid\":\"f830f98a-8e8b-4468-adf4-d6eab644987f\"},{\"content\":{\"connectorIds\":[\"Out1\",\"Out2\"],\"side\":\"RIGHT\"},\"type\":\"ConnectorPlacement.EquallySpacedRectSide\",\"uuid\":\"7e0d0116-b3ba-4668-b638-30d0f54ba087\"},{\"content\":{\"side\":\"TOP\"},\"type\":\"ConnectorPlacement.EquallySpacedRectSide\",\"uuid\":\"7b4146d3-46d2-45ca-8c34-b106f0d8cedd\"}]},\"type\":\"ConnectorPlacement.EquallySpacedConnector\",\"uuid\":\"3d911b2d-a78f-42ea-b869-5e09982d9f54\"}],\"packageUris\":[\"http://schema.mathworks.com/mf0/Connector/R2020b\"],\"version\":\"1.0\"}"
  CellQCSensor : Subsystem
      settings: PortSchema="{\"entries\":[{\"content\":{\"headerSize\":26,\"margin\":15,\"minimumSpacing\":25,\"sides\":[{\"content\":{\"connectorIds\":[\"In1\",\"In2\"]},\"type\":\"ConnectorPlacement.EquallySpacedRectSide\",\"uuid\":\"f830f98a-8e8b-4468-adf4-d6eab644987f\"},{\"content\":{\"connectorIds\":[\"Out1\",\"Out2\"],\"side\":\"RIGHT\"},\"type\":\"ConnectorPlacement.EquallySpacedRectSide\",\"uuid\":\"7e0d0116-b3ba-4668-b638-30d0f54ba087\"},{\"content\":{\"side\":\"TOP\"},\"type\":\"ConnectorPlacement.EquallySpacedRectSide\",\"uuid\":\"7b4146d3-46d2-45ca-8c34-b106f0d8cedd\"}]},\"type\":\"ConnectorPlacement.EquallySpacedConnector\",\"uuid\":\"3d911b2d-a78f-42ea-b869-5e09982d9f54\"}],\"packageUris\":[\"http://schema.mathworks.com/mf0/Connector/R2020b\"],\"version\":\"1.0\"}"
  Bus Element Out1 : Outport  PortName=sealedContainers
  Bus Element Out2 : Outport  Port=2  PortName=statusCell
  wires:
  Bus Element In1/1 -> CellPrepUnit/1(stagedIngredients)
  CellPrepUnit/1(preppedBatch) -> CellCookVat/1(preppedBatch)
  CellQCSensor/1(approvedSoup) -> CellPackager/1(approvedSoup)
  CellPrepUnit/2(statusPrep) -> CellController/2(statusPrep)
  CellQCSensor/2(statusQA) -> CellController/4(statusQA)
  CellPackager/1(sealedContainers) -> Bus Element Out1/1
  CellPackager/2(statusPack) -> CellController/5(statusPack)
  CellCookVat/1(cookedSoup) -> CellQCSensor/1(cookedSoup)
  CellCookVat/2(statusCook) -> CellController/3(statusCook)
  Bus Element In2/1 -> CellController/1(directive)
  CellController/1(cellDirective) -> CellPrepUnit/2(directive), CellPackager/2(directive), CellQCSensor/2(directive), CellCookVat/2(directive)
  CellController/2(statusCell) -> Bus Element Out2/1

== system PhysicalEverSimmer/IntakeAndStorage/AutoDock ==
  in_inboundCargo : Inport  PortName=inboundCargo  Element=flow_bps
  in_directive : Inport  Port=2  PortName=directive
  in_inboundCargoCap : Saturate  UpperLimit=0.0833333333333  LowerLimit=0
  receivedIngredients_c1 : Constant  Value=0
  receivedIngredients_c2 : Constant  Value=0
  receivedIngredients_c3 : Constant  Value=4
  statusReceive_c1 : Constant
  statusReceive_c2 : Constant
  statusReceive_c3 : Constant  Value=0
  statusReceive_c4 : Constant  Value=12
  statusReceive_h : Constant
  out_receivedIngredients : Outport  PortName=receivedIngredients  Element=palletId
  receivedIngredients_el2 : Outport  PortName=receivedIngredients  Element=mass_kg
  receivedIngredients_el3 : Outport  PortName=receivedIngredients  Element=temp_C
  receivedIngredients_el4 : Outport  PortName=receivedIngredients  Element=flow_bps
  out_statusReceive : Outport  Port=2  PortName=statusReceive  Element=unitId
  statusReceive_el2 : Outport  Port=2  PortName=statusReceive  Element=opState
  statusReceive_el3 : Outport  Port=2  PortName=statusReceive  Element=faultCode
  statusReceive_el4 : Outport  Port=2  PortName=statusReceive  Element=power_kW
  statusReceive_el5 : Outport  Port=2  PortName=statusReceive  Element=health
  wires:
  in_inboundCargo/1 -> in_inboundCargoCap/1
  statusReceive_h/1 -> statusReceive_el5/1
  receivedIngredients_c3/1 -> receivedIngredients_el3/1
  statusReceive_c1/1 -> out_statusReceive/1
  receivedIngredients_c2/1 -> receivedIngredients_el2/1
  statusReceive_c4/1 -> statusReceive_el4/1
  statusReceive_c2/1 -> statusReceive_el2/1
  receivedIngredients_c1/1 -> out_receivedIngredients/1
  statusReceive_c3/1 -> statusReceive_el3/1
  in_inboundCargoCap/1 -> receivedIngredients_el4/1

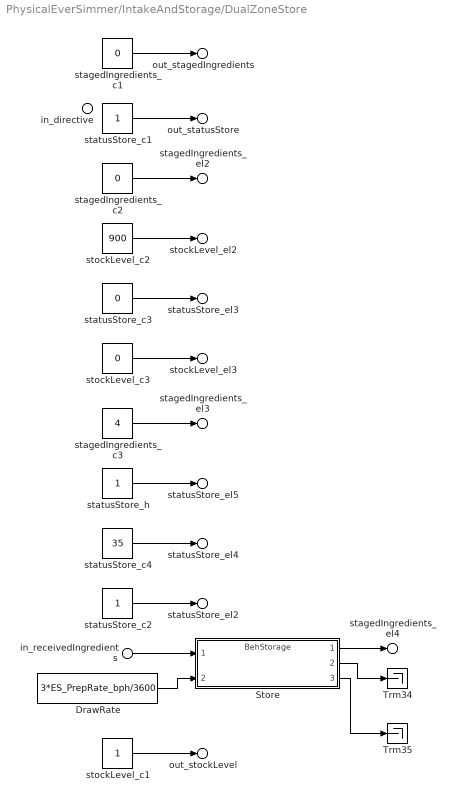
== system PhysicalEverSimmer/IntakeAndStorage/DualZoneStore ==
  in_receivedIngredients : Inport  PortName=receivedIngredients  Element=flow_bps
  in_directive : Inport  Port=2  PortName=directive  Element=setpoint
  DrawRate : Constant  Value=3*ES_PrepRate_bph/3600
  Store : ModelReference  ModelNameDialog=BehStorage  UsingDefaultArgumentValue=0,0  SimulationMode=Normal  ModelReferenceVersion=1.4
  Trm34 : Terminator
  Trm35 : Terminator
  stagedIngredients_c1 : Constant  Value=0
  stagedIngredients_c2 : Constant  Value=0
  stagedIngredients_c3 : Constant  Value=4
  statusStore_c1 : Constant
  statusStore_c2 : Constant
  statusStore_c3 : Constant  Value=0
  statusStore_c4 : Constant  Value=35
  statusStore_h : Constant
  stockLevel_c1 : Constant
  stockLevel_c2 : Constant  Value=900
  stockLevel_c3 : Constant  Value=0
  out_stagedIngredients : Outport  PortName=stagedIngredients  Element=palletId
  stagedIngredients_el2 : Outport  PortName=stagedIngredients  Element=mass_kg
  stagedIngredients_el3 : Outport  PortName=stagedIngredients  Element=temp_C
  stagedIngredients_el4 : Outport  PortName=stagedIngredients  Element=flow_bps
  out_stockLevel : Outport  Port=2  PortName=stockLevel  Element=itemId
  stockLevel_el2 : Outport  Port=2  PortName=stockLevel  Element=qty_units
  stockLevel_el3 : Outport  Port=2  PortName=stockLevel  Element=error_pct
  out_statusStore : Outport  Port=3  PortName=statusStore  Element=unitId
  statusStore_el2 : Outport  Port=3  PortName=statusStore  Element=opState
  statusStore_el3 : Outport  Port=3  PortName=statusStore  Element=faultCode
  statusStore_el4 : Outport  Port=3  PortName=statusStore  Element=power_kW
  statusStore_el5 : Outport  Port=3  PortName=statusStore  Element=health
  wires:
  stagedIngredients_c1/1 -> out_stagedIngredients/1
  statusStore_c1/1 -> out_statusStore/1
  statusStore_c3/1 -> statusStore_el3/1
  stockLevel_c2/1 -> stockLevel_el2/1
  stagedIngredients_c2/1 -> stagedIngredients_el2/1
  stagedIngredients_c3/1 -> stagedIngredients_el3/1
  stockLevel_c3/1 -> stockLevel_el3/1
  statusStore_h/1 -> statusStore_el5/1
  statusStore_c4/1 -> statusStore_el4/1
  Store/2 -> Trm34/1
  statusStore_c2/1 -> statusStore_el2/1
  in_receivedIngredients/1 -> Store/1
  DrawRate/1 -> Store/2
  stockLevel_c1/1 -> out_stockLevel/1
  Store/1 -> stagedIngredients_el4/1
  Store/3 -> Trm35/1

== system PhysicalEverSimmer/IntakeAndStorage/IntakeController ==
  in_directive : Inport  PortName=directive
  in_statusReceive : Inport  Port=2  PortName=statusReceive  Element=power_kW
  statusReceiveHlth : Inport  Port=2  PortName=statusReceive  Element=health
  in_statusStore : Inport  Port=3  PortName=statusStore  Element=power_kW
  statusStoreHlth : Inport  Port=3  PortName=statusStore  Element=health
  BayHealth : MinMax  Inputs=2
  BayPower : Sum
  HealthPad : Constant
  MemberHealth : Mux
  bayDirective_c1 : Constant  Value=0
  bayDirective_c2 : Constant  Value=0
  bayDirective_c3 : Constant
  bayStatus_c1 : Constant
  bayStatus_c2 : Constant
  bayStatus_c3 : Constant  Value=0
  out_bayDirective : Outport  PortName=bayDirective  Element=cmdType
  bayDirective_el2 : Outport  PortName=bayDirective  Element=targetId
  bayDirective_el3 : Outport  PortName=bayDirective  Element=setpoint
  out_bayStatus : Outport  Port=2  PortName=bayStatus  Element=unitId
  bayStatus_el2 : Outport  Port=2  PortName=bayStatus  Element=opState
  bayStatus_el3 : Outport  Port=2  PortName=bayStatus  Element=faultCode
  bayStatus_el4 : Outport  Port=2  PortName=bayStatus  Element=power_kW
  bayStatus_el5 : Outport  Port=2  PortName=bayStatus  Element=health
  bayStatus_el6 : Outport  Port=2  PortName=bayStatus  Element=lineHealth
  wires:
  bayStatus_c2/1 -> bayStatus_el2/1
  bayDirective_c3/1 -> bayDirective_el3/1
  statusReceiveHlth/1 -> BayHealth/1, MemberHealth/1
  bayStatus_c1/1 -> out_bayStatus/1
  bayDirective_c1/1 -> out_bayDirective/1
  bayStatus_c3/1 -> bayStatus_el3/1
  in_statusReceive/1 -> BayPower/1
  in_statusStore/1 -> BayPower/2
  HealthPad/1 -> MemberHealth/3, MemberHealth/4
  statusStoreHlth/1 -> BayHealth/2, MemberHealth/2
  bayDirective_c2/1 -> bayDirective_el2/1
  BayPower/1 -> bayStatus_el4/1
  MemberHealth/1 -> bayStatus_el6/1
  BayHealth/1 -> bayStatus_el5/1

== system PhysicalEverSimmer/IntakeAndStorage/SmartInventoryNet ==
  in_stockLevel : Inport  PortName=stockLevel
  inventoryStatus_c1 : Constant
  inventoryStatus_c2 : Constant  Value=900
  inventoryStatus_c3 : Constant  Value=0
  reorderRequest_c1 : Constant
  reorderRequest_c2 : Constant  Value=0
  reorderRequest_c3 : Constant  Value=0
  out_inventoryStatus : Outport  PortName=inventoryStatus  Element=itemId
  inventoryStatus_el2 : Outport  PortName=inventoryStatus  Element=qty_units
  inventoryStatus_el3 : Outport  PortName=inventoryStatus  Element=error_pct
  out_reorderRequest : Outport  Port=2  PortName=reorderRequest  Element=itemId
  reorderRequest_el2 : Outport  Port=2  PortName=reorderRequest  Element=qty_units
  reorderRequest_el3 : Outport  Port=2  PortName=reorderRequest  Element=error_pct
  wires:
  reorderRequest_c2/1 -> reorderRequest_el2/1
  reorderRequest_c3/1 -> reorderRequest_el3/1
  inventoryStatus_c1/1 -> out_inventoryStatus/1
  inventoryStatus_c3/1 -> inventoryStatus_el3/1
  reorderRequest_c1/1 -> out_reorderRequest/1
  inventoryStatus_c2/1 -> inventoryStatus_el2/1
